simulink model "model_sym_DC"  (R2014a)
settings: Solver=ode3  StartTime=0.0  StopTime=Tsim  FixedStep=Tp  RelTol=1e-3
values from neighbouring files (symbols this model uses):
  J = 0.32    [neural_observer_example_01.m]    (also in neural_observer_example_02.m; neural_observer_example_03b.m)
  kfi = 4.13    [neural_observer_example_01.m]    (also in neural_observer_example_02.m; neural_observer_example_03b.m)
  L = 7.85e-3    (= 0.00785)    [neural_observer_example_01.m]    (also in neural_observer_example_02.m; neural_observer_example_03b.m)
  R = 0.472    [neural_observer_example_01.m]    (also in neural_observer_example_02.m; neural_observer_example_03b.m)
settings Model: Creator=Jacek  LastModifiedBy=Jacek
settings DataIOCC: LimitDataPoints=off

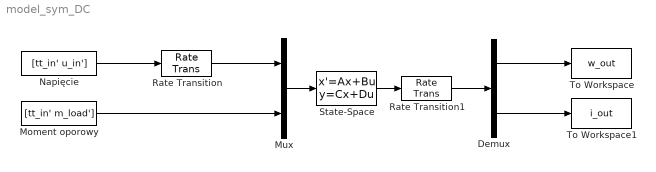
== system model_sym_DC ==
  Demux : Demux  Outputs=2
  Moment oporowy : FromWorkspace  VariableName=[tt_in' m_load']  SampleTime=0
  Mux : Mux  Inputs=2
  Napięcie : FromWorkspace  VariableName=[tt_in' u_in']  SampleTime=0
  Rate Transition : RateTransition
  Rate Transition1 : RateTransition
  State-Space : StateSpace  A=[-R/L -kfi/L; kfi/J 0]  B=[1/L 0; 0 -1/J]  C=[0 1; 1 0]  D=[0 0; 0 0]  X0=0
  To Workspace : ToWorkspace  VariableName=w_out  SampleTime=-1
  To Workspace1 : ToWorkspace  VariableName=i_out  SampleTime=-1
  wires:
  Napięcie/1 -> Rate Transition/1
  Rate Transition/1 -> Mux/1
  Moment oporowy/1 -> Mux/2
  Mux/1 -> State-Space/1
  State-Space/1 -> Rate Transition1/1
  Rate Transition1/1 -> Demux/1
  Demux/1 -> To Workspace/1
  Demux/2 -> To Workspace1/1
